simulink model "observer_for_disturbance"  (R2023b)
settings: Solver=FixedStepAuto  StartTime=0.0  StopTime=15.0  FixedStep=0.001  RelTol=1e-3
values from neighbouring files (symbols this model uses):
  Ae = [A, B; zeros(1,3)]    [observer_for_disturbance_par.m]
  Be = [B; 0]    [observer_for_disturbance_par.m]
  Ce = [C, zeros(2,1)]    [observer_for_disturbance_par.m]
  L_des = place(Ae',Ce',lambda_des)'    [observer_for_disturbance_par.m]
  x0 = [2; 200; 0]    [observer_for_disturbance_par.m]    (also in openloop_control_par.m = [ 2 ; 200 ]; state_feedback_around_eq_par.m = [2; 200])
settings Model: Creator=peterparker  LastModifiedBy=peterparker

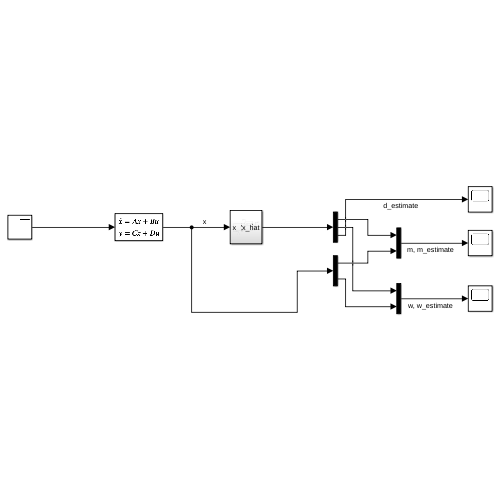
[thumbnail: Simulink's stored preview of the top-level diagram]
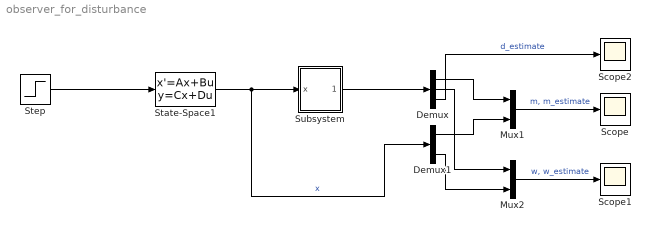
== system observer_for_disturbance ==
  Demux : Demux  Outputs=3
  Demux1 : Demux  Outputs=2
  Mux1 : Mux  Inputs=2
  Mux2 : Mux  Inputs=2
  Scope : Scope
  Scope1 : Scope
  Scope2 : Scope
  State-Space1 : StateSpace  A=Ae  B=Be  C=Ce  D=zeros(2,1)  InitialCondition=x0
  Step : Step  Time=5  After=10  SampleTime=0
  Subsystem : Subsystem
  wires:
  Subsystem/1(x_hat) -> Demux/1
  State-Space1/1 -> Demux1/1, Subsystem/1(x)  "x"
  Step/1 -> State-Space1/1
  Demux/1 -> Mux1/1
  Demux1/1 -> Mux1/2
  Demux/2 -> Mux2/1
  Demux1/2 -> Mux2/2
  Mux1/1 -> Scope/1  "m, m_estimate"
  Mux2/1 -> Scope1/1  "w, w_estimate"
  Demux/3 -> Scope2/1  "d_estimate"

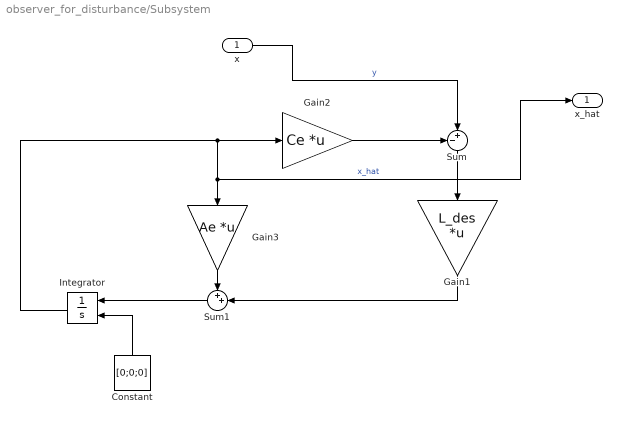
== system observer_for_disturbance/Subsystem ==
  x : Inport
  Constant : Constant  Value=[0;0;0]
  Gain1 : Gain  Gain=L_des  Multiplication=Matrix(K*u) (u vector)
  Gain2 : Gain  Gain=Ce  Multiplication=Matrix(K*u) (u vector)
  Gain3 : Gain  Gain=Ae  Multiplication=Matrix(K*u) (u vector)
  Integrator : Integrator  InitialConditionSource=external
  Sum : Sum  Inputs=-+|
  Sum1 : Sum  Inputs=++|
  x_hat : Outport
  wires:
  x/1 -> Sum/2  "y"
  Sum1/1 -> Integrator/1
  Gain2/1 -> Sum/1
  Gain1/1 -> Sum1/2
  Gain3/1 -> Sum1/1
  Constant/1 -> Integrator/2
  Sum/1 -> Gain1/1
  Integrator/1 -> x_hat/1, Gain3/1, Gain2/1  "x_hat"
